simulink model "SimulinkBallbotModel"  (R2017a)
settings: Solver=FixedStepDiscrete  StartTime=0.0  StopTime=10  RelTol=1e-3
libraries: simulink x2
settings Model: FPTRunName=Active  ExtModeTrigDuration=2  Creator=Christopher  LastModifiedBy=Christopher
settings DataIOCC: LimitDataPoints=on  SaveFormat=Array  DSMLogging=off
settings OptimizationCC: DefaultParameterBehavior=Inlined  UseDivisionForNetSlopeComputation=on  UseFloatMulNetSlope=on  InlineInvariantSignals=on  PassReuseOutputArgsAs=Individual arguments  ExpressionDepthLimit=2147483647  ZeroExternalMemoryAtStartup=off  ZeroInternalMemoryAtStartup=off  NoFixptDivByZeroProtection=on  EfficientFloat2IntCast=on  LifeSpan=1  MaxStackSize=64  OptimizeBlockOrder=speed
settings DebuggingCC: UnderspecifiedInitializationDetection=Classic  MergeDetectMultiDrivingBlocksExec=none  ParameterOverflowMsg=warning  ParameterPrecisionLossMsg=none  ParameterTunabilityLossMsg=error  FcnCallInpInsideContextMsg=warning  AllowSymbolicDim=off  StateNameClashWarn=warning  SFUnexpectedBacktrackingDiag=warning  SFNoUnconditionalDefaultTransitionDiag=warning  SFExecutionAtInitializationDiag=none
settings HardwareCC: ProdBitPerInt=16  ProdBitPerPointer=16  ProdBitPerSizeT=16  ProdBitPerPtrDiffT=16  ProdLargestAtomicFloat=None  ProdWordSize=8  ProdHWDeviceType=Atmel->AVR
settings ModelReferenceCC: PropagateSignalLabelsOutOfModel=off
settings SFSimCC: MATLABDynamicMemAlloc=off
settings RTWCC: SystemTargetFile=ert.tlc  HardwareBoard=Arduino Mega 2560  TLCOptions=-aInlineSetEventsForThisBaseRateFcn=TLC_FALSE -aSuppressMultiTaskScheduler=TLC_FALSE -aRateBasedStepFcn=1  GenCodeOnly=on  TemplateMakefile=ert_default_tmf  Description=Embedded Coder  GenerateReport=on  RTWVerbose=off  Toolchain=Arduino AVR  BuildConfiguration=Faster Runs  IncludeHyperlinkInReport=on  LaunchReport=on  GenerateTraceInfo=on  GenerateTraceReport=on  GenerateTraceReportSl=on  GenerateTraceReportSf=on  GenerateTraceReportEml=on  GenerateCodeMetricsReport=on
settings CodeAppCC: ForceParamTrailComments=on  IgnoreCustomStorageClasses=off  OperatorAnnotations=on  SimulinkDataObjDesc=on  SFDataObjDesc=on  MATLABFcnDesc=on  CustomSymbolStrGlobalVar=rt$N$M  CustomSymbolStrType=$N$M  CustomSymbolStrFcn=$N$M$F  CustomSymbolStrMacro=$N$M  InsertBlockDesc=on  MATLABSourceComments=on
settings ERTTargetCC: TargetLangStandard=C99 (ISO)  IncludeMdlTerminateFcn=off  CombineSignalStateStructs=on  SuppressErrorStatus=on  SupportAbsoluteTime=off  SupportNonFinite=off  SupportComplex=off  InlinedParameterPlacement=NonHierarchical  ERTFilePackagingFormat=CompactWithDataFile
settings ConfigComp: CovMetricSettings=dw  CovHtmlReporting=on  CovSaveCumulativeToWorkspaceVar=on  CovSaveSingleToWorkspaceVar=on  CovExternalEMLEnable=off  CovSFcnEnable=off

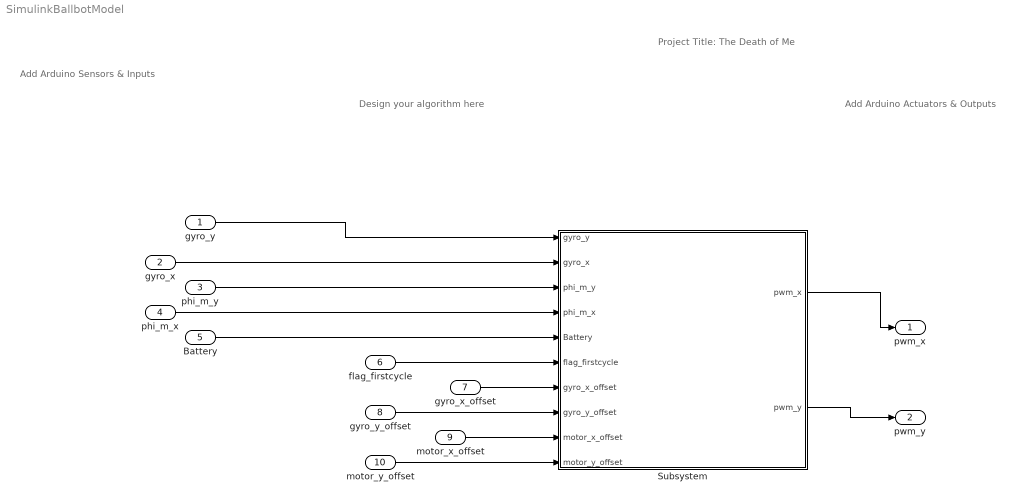
== system SimulinkBallbotModel ==
  note: Project Title: The Death of Me
  note: Add Arduino Sensors & Inputs
  note: Design your algorithm here
  note: Add Arduino Actuators & Outputs
  gyro_y : Inport  OutDataTypeStr=uint16
  gyro_x : Inport  Port=2  OutDataTypeStr=uint16
  phi_m_y : Inport  Port=3  OutDataTypeStr=int32
  phi_m_x : Inport  Port=4  OutDataTypeStr=int32
  Battery : Inport  Port=5  OutDataTypeStr=single
  flag_firstcycle : Inport  Port=6  OutDataTypeStr=boolean
  gyro_x_offset : Inport  Port=7  OutDataTypeStr=single
  gyro_y_offset : Inport  Port=8  OutDataTypeStr=single
  motor_x_offset : Inport  Port=9  OutDataTypeStr=single
  motor_y_offset : Inport  Port=10  OutDataTypeStr=single
  Subsystem : Subsystem
  pwm_x : Outport  OutDataTypeStr=int8
  pwm_y : Outport  Port=2  OutDataTypeStr=int8
  wires:
  phi_m_x/1 -> Subsystem/4(phi_m_x)
  Battery/1 -> Subsystem/5(Battery)
  Subsystem/1(pwm_x) -> pwm_x/1
  Subsystem/2(pwm_y) -> pwm_y/1
  phi_m_y/1 -> Subsystem/3(phi_m_y)
  gyro_x/1 -> Subsystem/2(gyro_x)
  gyro_y/1 -> Subsystem/1(gyro_y)
  flag_firstcycle/1 -> Subsystem/6(flag_firstcycle)
  gyro_x_offset/1 -> Subsystem/7(gyro_x_offset)
  gyro_y_offset/1 -> Subsystem/8(gyro_y_offset)
  motor_x_offset/1 -> Subsystem/9(motor_x_offset)
  motor_y_offset/1 -> Subsystem/10(motor_y_offset)

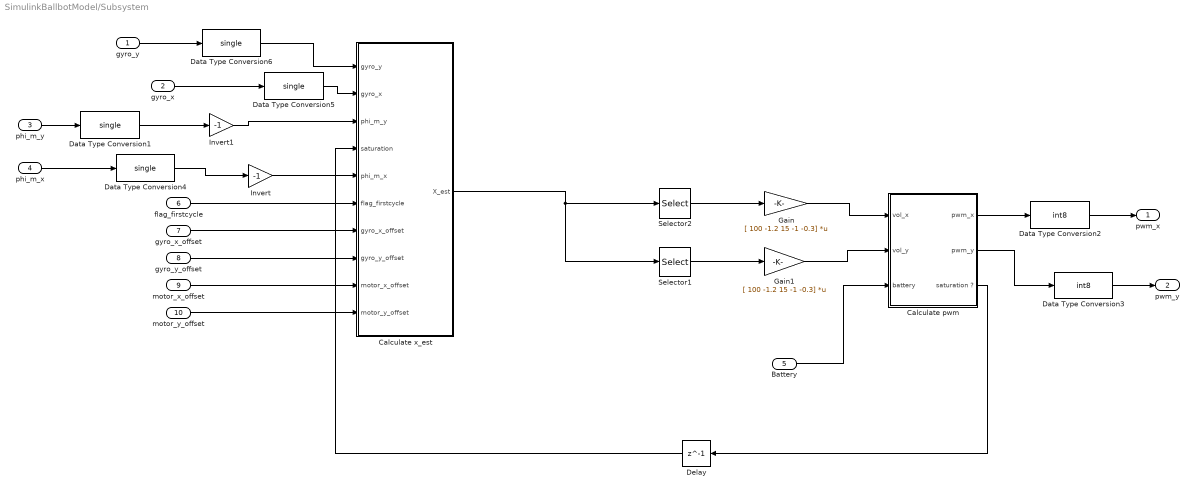
== system SimulinkBallbotModel/Subsystem ==
  gyro_y : Inport
  gyro_x : Inport  Port=2
  phi_m_y : Inport  Port=3  OutDataTypeStr=int32
  phi_m_x : Inport  Port=4  OutDataTypeStr=int32
  Battery : Inport  Port=5  OutDataTypeStr=single
  flag_firstcycle : Inport  Port=6
  gyro_x_offset : Inport  Port=7
  gyro_y_offset : Inport  Port=8
  motor_x_offset : Inport  Port=9
  motor_y_offset : Inport  Port=10
  Calculate pwm : Subsystem
  Calculate x_est : Subsystem
  Data Type Conversion{1,4..6} (4 alike) : DataTypeConversion  OutDataTypeStr=single  RndMeth=Simplest
  Data Type Conversion2 : DataTypeConversion  OutDataTypeStr=int8  RndMeth=Simplest
  Data Type Conversion3 : DataTypeConversion  OutDataTypeStr=int8  RndMeth=Simplest
  Delay : Delay  DelayLength=1  InitialCondition=0
  Gain : Gain  Gain=[ 100 -1.2 15 -1 -0.3]  Multiplication=Matrix(K*u) (u vector)  OutDataTypeStr=single
  Gain1 : Gain  Gain=[ 100 -1.2 15 -1 -0.3]  Multiplication=Matrix(K*u) (u vector)  OutDataTypeStr=single
  Invert : Gain  Gain=-1  OutDataTypeStr=single
  Invert1 : Gain  Gain=-1  OutDataTypeStr=single
  Selector1 : Selector  IndexMode=Zero-based  InputPortWidth=10  IndexOptions=Starting index (dialog)  Indices=5  OutputSizes=5
  Selector2 : Selector  IndexMode=Zero-based  InputPortWidth=10  IndexOptions=Starting index (dialog)  Indices=0  OutputSizes=5
  pwm_x : Outport  OutDataTypeStr=int8
  pwm_y : Outport  Port=2  OutDataTypeStr=int8
  wires:
  Gain1/1 -> Calculate pwm/2(vol_y)
  Calculate x_est/1(X_est) -> Selector1/1, Selector2/1
  Gain/1 -> Calculate pwm/1(vol_x)
  gyro_x/1 -> Data Type Conversion5/1
  Calculate pwm/1(pwm_x) -> Data Type Conversion2/1
  phi_m_x/1 -> Data Type Conversion4/1
  Delay/1 -> Calculate x_est/4(saturation)
  Calculate pwm/2(pwm_y) -> Data Type Conversion3/1
  phi_m_y/1 -> Data Type Conversion1/1
  Battery/1 -> Calculate pwm/3(battery)
  Selector2/1 -> Gain/1
  Calculate pwm/3(saturation ?) -> Delay/1
  Selector1/1 -> Gain1/1
  gyro_y/1 -> Data Type Conversion6/1
  flag_firstcycle/1 -> Calculate x_est/6(flag_firstcycle)
  gyro_x_offset/1 -> Calculate x_est/7(gyro_x_offset)
  gyro_y_offset/1 -> Calculate x_est/8(gyro_y_offset)
  motor_x_offset/1 -> Calculate x_est/9(motor_x_offset)
  motor_y_offset/1 -> Calculate x_est/10(motor_y_offset)
  Data Type Conversion2/1 -> pwm_x/1
  Data Type Conversion3/1 -> pwm_y/1
  Data Type Conversion6/1 -> Calculate x_est/1(gyro_y)
  Data Type Conversion5/1 -> Calculate x_est/2(gyro_x)
  Data Type Conversion1/1 -> Invert1/1
  Data Type Conversion4/1 -> Invert/1
  Invert/1 -> Calculate x_est/5(phi_m_x)
  Invert1/1 -> Calculate x_est/3(phi_m_y)

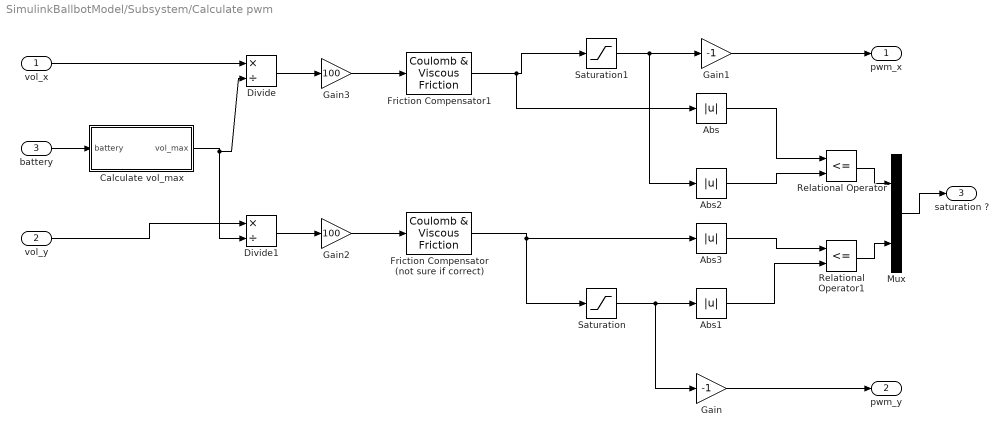
== system SimulinkBallbotModel/Subsystem/Calculate pwm ==
  vol_x : Inport  OutDataTypeStr=single
  vol_y : Inport  Port=2  OutDataTypeStr=single
  battery : Inport  Port=3  OutDataTypeStr=single
  Abs{,1..3} (4 alike) : Abs
  Calculate vol_max : Subsystem
  Divide : Product  Inputs=*/  OutDataTypeStr=single
  Divide1 : Product  Inputs=*/  OutDataTypeStr=single
  Friction Compensator (not sure if correct) : simulink/Discontinuities/Coulomb & Viscous Friction  offset=0  gain=1
      settings: SourceProductName=Simulink
  Friction Compensator1 : simulink/Discontinuities/Coulomb & Viscous Friction  offset=0  gain=1
      settings: SourceProductName=Simulink
  Gain : Gain  Gain=-1  OutDataTypeStr=single  RndMeth=Simplest
  Gain1 : Gain  Gain=-1  OutDataTypeStr=single  RndMeth=Simplest
  Gain2 : Gain  Gain=100  OutDataTypeStr=single
  Gain3 : Gain  Gain=100  OutDataTypeStr=single
  Mux : Mux  Inputs=2
  Relational Operator : RelationalOperator  Operator=<=  OutDataTypeStr=boolean  RndMeth=Simplest
  Relational Operator1 : RelationalOperator  Operator=<=  OutDataTypeStr=boolean  RndMeth=Simplest
  Saturation : Saturate  UpperLimit=100  LowerLimit=-100  OutDataTypeStr=single
  Saturation1 : Saturate  UpperLimit=100  LowerLimit=-100  OutDataTypeStr=single
  pwm_x : Outport  OutDataTypeStr=single
  pwm_y : Outport  Port=2  OutDataTypeStr=single
  saturation ? : Outport  Port=3  OutDataTypeStr=boolean
  wires:
  battery/1 -> Calculate vol_max/1(battery)
  Gain/1 -> pwm_y/1
  Gain1/1 -> pwm_x/1
  Mux/1 -> saturation ?/1
  Relational Operator/1 -> Mux/1
  Relational Operator1/1 -> Mux/2
  Abs3/1 -> Relational Operator1/1
  Abs1/1 -> Relational Operator1/2
  Abs2/1 -> Relational Operator/2
  Abs/1 -> Relational Operator/1
  Saturation/1 -> Gain/1, Abs1/1
  Saturation1/1 -> Abs2/1, Gain1/1
  vol_x/1 -> Divide/1
  vol_y/1 -> Divide1/1
  Calculate vol_max/1(vol_max) -> Divide/2, Divide1/2
  Divide/1 -> Gain3/1
  Divide1/1 -> Gain2/1
  Gain2/1 -> Friction Compensator (not sure if correct)/1
  Gain3/1 -> Friction Compensator1/1
  Friction Compensator1/1 -> Abs/1, Saturation1/1
  Friction Compensator (not sure if correct)/1 -> Abs3/1, Saturation/1

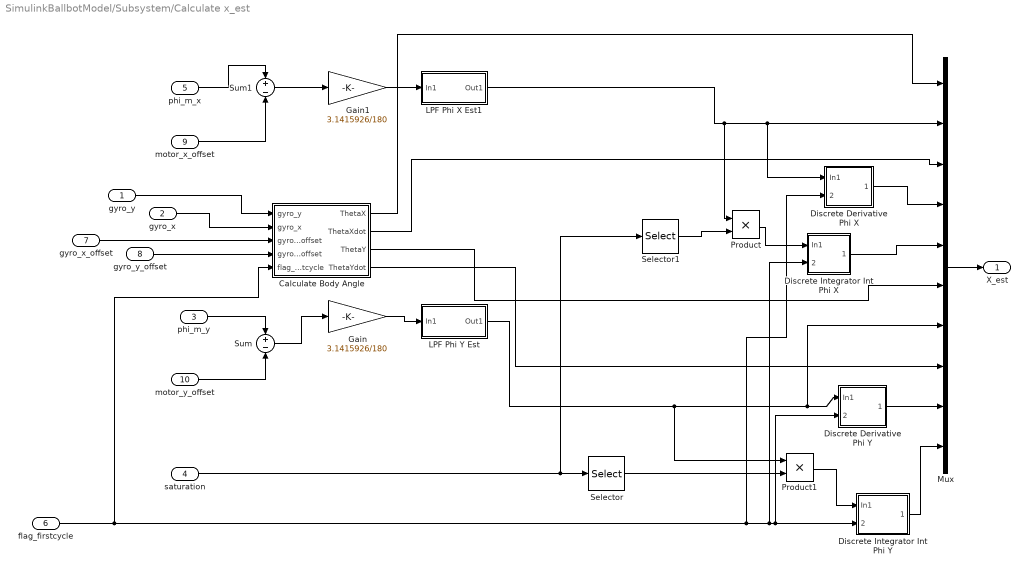
== system SimulinkBallbotModel/Subsystem/Calculate x_est ==
  gyro_y : Inport  OutDataTypeStr=single
  gyro_x : Inport  Port=2  OutDataTypeStr=single
  phi_m_y : Inport  Port=3
  saturation : Inport  Port=4  OutDataTypeStr=boolean
  phi_m_x : Inport  Port=5
  flag_firstcycle : Inport  Port=6
  gyro_x_offset : Inport  Port=7
  gyro_y_offset : Inport  Port=8
  motor_x_offset : Inport  Port=9
  motor_y_offset : Inport  Port=10
  Calculate Body Angle : Subsystem
  Discrete Derivative Phi X : Subsystem  TreatAsAtomicUnit=on
  Discrete Derivative Phi Y : Subsystem  TreatAsAtomicUnit=on
  Discrete Integrator Int Phi X : Subsystem  TreatAsAtomicUnit=on
  Discrete Integrator Int Phi Y : Subsystem  TreatAsAtomicUnit=on
  Gain : Gain  Gain=3.1415926/180  OutDataTypeStr=single
  Gain1 : Gain  Gain=3.1415926/180  OutDataTypeStr=single
  LPF Phi X Est1 : Subsystem
  LPF Phi Y Est : Subsystem
  Mux : Mux  Inputs=10
  Product : Product
  Product1 : Product  OutDataTypeStr=single
  Selector : Selector  IndexMode=Zero-based  InputPortWidth=2  IndexOptions=Starting index (dialog)  Indices=1  OutputSizes=1
  Selector1 : Selector  IndexMode=Zero-based  InputPortWidth=2  IndexOptions=Starting index (dialog)  Indices=0  OutputSizes=1
  Sum : Sum  Inputs=+-
  Sum1 : Sum  Inputs=+-  AccumDataTypeStr=uint8
  X_est : Outport  OutDataTypeStr=single
  wires:
  Mux/1 -> X_est/1
  Product/1 -> Discrete Integrator Int Phi X/1(In1)
  Discrete Integrator Int Phi Y/1(Out1) -> Mux/10
  phi_m_y/1 -> Sum/1
  Discrete Integrator Int Phi X/1(Out1) -> Mux/5
  saturation/1 -> Selector1/1, Selector/1
  Product1/1 -> Discrete Integrator Int Phi Y/1(In1)
  Discrete Derivative Phi Y/1(Out1) -> Mux/9
  Calculate Body Angle/4(ThetaYdot) -> Mux/8
  Sum/1 -> Gain/1
  LPF Phi Y Est/1(Out1) -> Product1/1, Mux/7, Discrete Derivative Phi Y/1(In1)
  Gain1/1 -> LPF Phi X Est1/1(In1)
  Sum1/1 -> Gain1/1
  Discrete Derivative Phi X/1(Out1) -> Mux/4
  Selector1/1 -> Product/2
  Selector/1 -> Product1/2
  Gain/1 -> LPF Phi Y Est/1(In1)
  gyro_x/1 -> Calculate Body Angle/2(gyro_x)
  phi_m_x/1 -> Sum1/1
  Calculate Body Angle/2(ThetaXdot) -> Mux/3
  Calculate Body Angle/3(ThetaY) -> Mux/6
  gyro_y/1 -> Calculate Body Angle/1(gyro_y)
  LPF Phi X Est1/1(Out1) -> Product/1, Discrete Derivative Phi X/1(In1), Mux/2
  Calculate Body Angle/1(ThetaX) -> Mux/1
  motor_x_offset/1 -> Sum1/2
  motor_y_offset/1 -> Sum/2
  flag_firstcycle/1 -> Calculate Body Angle/5(flag_firstcycle), Discrete Integrator Int Phi X/2(flag_firstcycle), Discrete Derivative Phi Y/2(flag_firstcycle), Discrete Integrator Int Phi Y/2(flag_firstcycle), Discrete Derivative Phi X/2(flag_firstcycle)
  gyro_x_offset/1 -> Calculate Body Angle/3(gyro_x_offset)
  gyro_y_offset/1 -> Calculate Body Angle/4(gyro_y_offset)

== system SimulinkBallbotModel/Subsystem/Calculate pwm/Calculate vol_max ==
  battery : Inport
  Constant : Constant  Value=0.625  OutDataTypeStr=single
  Gain : Gain  Gain=.001089  OutDataTypeStr=single  RndMeth=Simplest
  Sum : Sum  Inputs=+-
  vol_max : Outport
  wires:
  battery/1 -> Gain/1
  Gain/1 -> Sum/1
  Constant/1 -> Sum/2
  Sum/1 -> vol_max/1

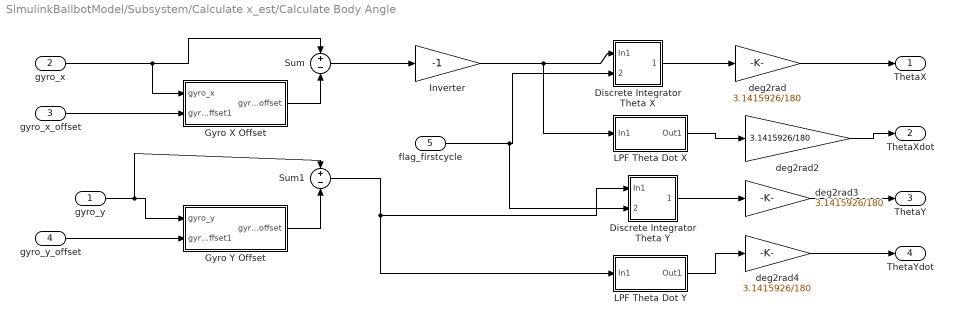
== system SimulinkBallbotModel/Subsystem/Calculate x_est/Calculate Body Angle ==
  gyro_y : Inport  OutDataTypeStr=single
  gyro_x : Inport  Port=2  OutDataTypeStr=single
  gyro_x_offset : Inport  Port=3  OutDataTypeStr=single
  gyro_y_offset : Inport  Port=4  OutDataTypeStr=single
  flag_firstcycle : Inport  Port=5  OutDataTypeStr=boolean
  Discrete Integrator Theta Y : Subsystem  TreatAsAtomicUnit=on
  Discrete Integrator Theta X : Subsystem  TreatAsAtomicUnit=on
  Gyro X Offset : Subsystem
  Gyro Y Offset : Subsystem
  Inverter : Gain  Gain=-1  OutDataTypeStr=single
  LPF Theta Dot X : Subsystem
  LPF Theta Dot Y : Subsystem
  Sum : Sum  Inputs=+-
  Sum1 : Sum  Inputs=+-
  deg2rad{,2..4} (4 alike) : Gain  Gain=3.1415926/180  OutDataTypeStr=single
  ThetaX : Outport  OutDataTypeStr=single
  ThetaXdot : Outport  Port=2  OutDataTypeStr=single
  ThetaY : Outport  Port=3  OutDataTypeStr=single
  ThetaYdot : Outport  Port=4  OutDataTypeStr=single
  wires:
  deg2rad/1 -> ThetaX/1
  deg2rad4/1 -> ThetaYdot/1
  deg2rad3/1 -> ThetaY/1
  deg2rad2/1 -> ThetaXdot/1
  Gyro Y Offset/1(gyro_y_offset) -> Sum1/2
  Sum/1 -> Inverter/1
  Gyro X Offset/1(gyro_x_offset) -> Sum/2
  Discrete Integrator Theta X/1(Out1) -> deg2rad/1
  Discrete Integrator Theta Y/1(Out1) -> deg2rad3/1
  LPF Theta Dot X/1(Out1) -> deg2rad2/1
  LPF Theta Dot Y/1(Out1) -> deg2rad4/1
  Sum1/1 -> Discrete Integrator Theta Y/1(In1), LPF Theta Dot Y/1(In1)
  Inverter/1 -> LPF Theta Dot X/1(In1), Discrete Integrator Theta X/1(In1)
  gyro_x_offset/1 -> Gyro X Offset/2(gyro_x_offset1)
  gyro_y_offset/1 -> Gyro Y Offset/2(gyro_y_offset1)
  flag_firstcycle/1 -> Discrete Integrator Theta Y/2(flag_firstcycle), Discrete Integrator Theta X/2(flag_firstcycle)
  gyro_x/1 -> Gyro X Offset/1(gyro_x), Sum/1
  gyro_y/1 -> Sum1/1, Gyro Y Offset/1(gyro_y)

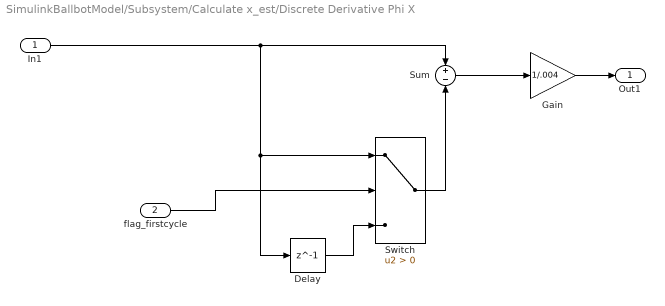
== system SimulinkBallbotModel/Subsystem/Calculate x_est/Discrete Derivative Phi X ==
  In1 : Inport
  flag_firstcycle : Inport  Port=2  OutDataTypeStr=boolean
  Delay : Delay  DelayLength=1  InitialCondition=0
  Gain : Gain  Gain=1/.004  OutDataTypeStr=single
  Sum : Sum  Inputs=+-
  Switch : Switch  Criteria=u2 > Threshold  OutDataTypeStr=single
  Out1 : Outport  OutDataTypeStr=single
  wires:
  Gain/1 -> Out1/1
  Switch/1 -> Sum/2
  In1/1 -> Delay/1, Switch/1, Sum/1
  Sum/1 -> Gain/1
  Delay/1 -> Switch/3
  flag_firstcycle/1 -> Switch/2

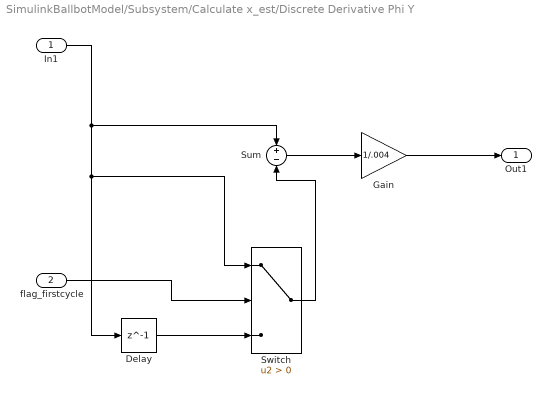
== system SimulinkBallbotModel/Subsystem/Calculate x_est/Discrete Derivative Phi Y ==
  In1 : Inport  OutDataTypeStr=single
  flag_firstcycle : Inport  Port=2
  Delay : Delay  DelayLength=1  InitialCondition=0
  Gain : Gain  Gain=1/.004  OutDataTypeStr=single
  Sum : Sum  Inputs=+-
  Switch : Switch  Criteria=u2 > Threshold  OutDataTypeStr=single
  Out1 : Outport  OutDataTypeStr=single
  wires:
  Sum/1 -> Gain/1
  Gain/1 -> Out1/1
  In1/1 -> Delay/1, Switch/1, Sum/1
  Delay/1 -> Switch/3
  Switch/1 -> Sum/2
  flag_firstcycle/1 -> Switch/2

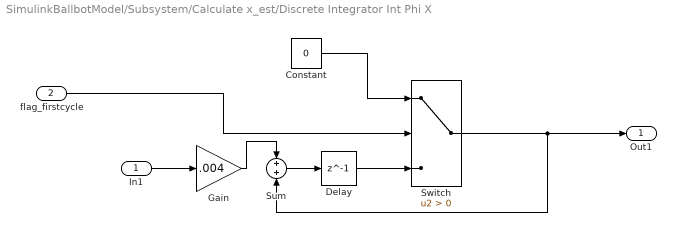
== system SimulinkBallbotModel/Subsystem/Calculate x_est/Discrete Integrator Int Phi X ==
  In1 : Inport  OutDataTypeStr=single
  flag_firstcycle : Inport  Port=2
  Constant : Constant  Value=0  OutDataTypeStr=single
  Delay : Delay  DelayLength=1  InitialCondition=0
  Gain : Gain  Gain=.004  OutDataTypeStr=single  RndMeth=Simplest
  Sum : Sum
  Switch : Switch  Criteria=u2 > Threshold  OutDataTypeStr=single
  Out1 : Outport  OutDataTypeStr=single
  wires:
  flag_firstcycle/1 -> Switch/2
  Delay/1 -> Switch/3
  In1/1 -> Gain/1
  Gain/1 -> Sum/1
  Sum/1 -> Delay/1
  Switch/1 -> Sum/2, Out1/1
  Constant/1 -> Switch/1

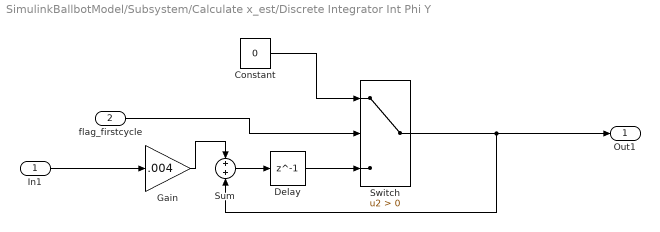
== system SimulinkBallbotModel/Subsystem/Calculate x_est/Discrete Integrator Int Phi Y ==
  In1 : Inport  OutDataTypeStr=single
  flag_firstcycle : Inport  Port=2  OutDataTypeStr=boolean
  Constant : Constant  Value=0  OutDataTypeStr=single
  Delay : Delay  DelayLength=1  InitialCondition=0
  Gain : Gain  Gain=.004  OutDataTypeStr=single  RndMeth=Simplest
  Sum : Sum
  Switch : Switch  Criteria=u2 > Threshold  OutDataTypeStr=single
  Out1 : Outport  OutDataTypeStr=single
  wires:
  Switch/1 -> Sum/2, Out1/1
  Delay/1 -> Switch/3
  flag_firstcycle/1 -> Switch/2
  Sum/1 -> Delay/1
  Constant/1 -> Switch/1
  Gain/1 -> Sum/1
  In1/1 -> Gain/1

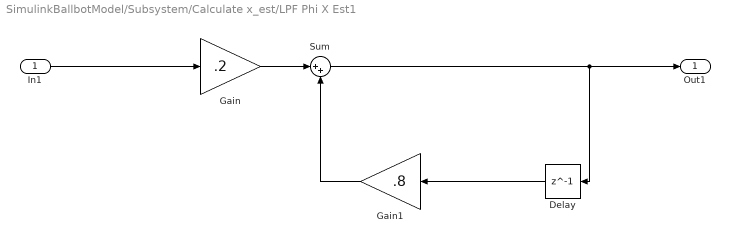
== system SimulinkBallbotModel/Subsystem/Calculate x_est/LPF Phi X Est1 ==
  In1 : Inport  OutDataTypeStr=single
  Delay : Delay  DelayLength=1  InitialCondition=0
  Gain : Gain  Gain=.2  OutDataTypeStr=single
  Gain1 : Gain  Gain=.8  OutDataTypeStr=single
  Sum : Sum  Inputs=|++
  Out1 : Outport  OutDataTypeStr=single
  wires:
  In1/1 -> Gain/1
  Gain1/1 -> Sum/2
  Gain/1 -> Sum/1
  Sum/1 -> Delay/1, Out1/1
  Delay/1 -> Gain1/1

== system SimulinkBallbotModel/Subsystem/Calculate x_est/LPF Phi Y Est ==
  In1 : Inport
  Delay : Delay  DelayLength=1  InitialCondition=0
  Gain : Gain  Gain=.2  OutDataTypeStr=single
  Gain1 : Gain  Gain=.8  OutDataTypeStr=single
  Sum : Sum  Inputs=|++
  Out1 : Outport  OutDataTypeStr=single
  wires:
  Sum/1 -> Out1/1, Delay/1
  Gain1/1 -> Sum/2
  Delay/1 -> Gain1/1
  Gain/1 -> Sum/1
  In1/1 -> Gain/1

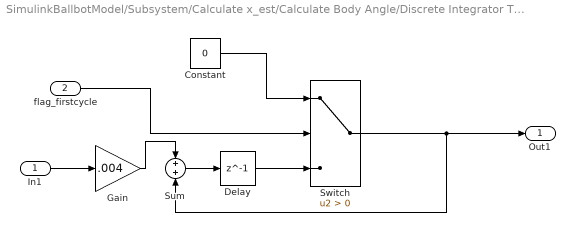
== system SimulinkBallbotModel/Subsystem/Calculate x_est/Calculate Body Angle/Discrete Integrator Theta Y ==
  In1 : Inport  OutDataTypeStr=single
  flag_firstcycle : Inport  Port=2  OutDataTypeStr=boolean
  Constant : Constant  Value=0  OutDataTypeStr=single
  Delay : Delay  DelayLength=1  InitialCondition=0
  Gain : Gain  Gain=.004  OutDataTypeStr=single
  Sum : Sum
  Switch : Switch  Criteria=u2 > Threshold  OutDataTypeStr=single
  Out1 : Outport  OutDataTypeStr=single
  wires:
  flag_firstcycle/1 -> Switch/2
  Delay/1 -> Switch/3
  In1/1 -> Gain/1
  Gain/1 -> Sum/1
  Sum/1 -> Delay/1
  Switch/1 -> Sum/2, Out1/1
  Constant/1 -> Switch/1

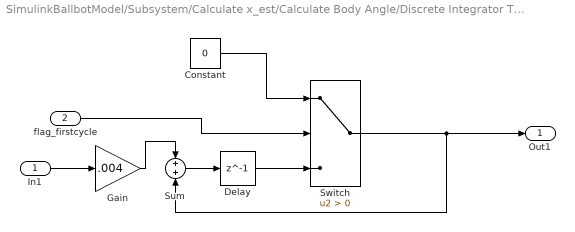
== system SimulinkBallbotModel/Subsystem/Calculate x_est/Calculate Body Angle/Discrete Integrator Theta X ==
  In1 : Inport
  flag_firstcycle : Inport  Port=2  OutDataTypeStr=boolean
  Constant : Constant  Value=0  OutDataTypeStr=single
  Delay : Delay  DelayLength=1  InitialCondition=0
  Gain : Gain  Gain=.004  OutDataTypeStr=single
  Sum : Sum
  Switch : Switch  Criteria=u2 > Threshold  OutDataTypeStr=single
  Out1 : Outport  OutDataTypeStr=single
  wires:
  flag_firstcycle/1 -> Switch/2
  Delay/1 -> Switch/3
  In1/1 -> Gain/1
  Gain/1 -> Sum/1
  Sum/1 -> Delay/1
  Switch/1 -> Sum/2, Out1/1
  Constant/1 -> Switch/1

== system SimulinkBallbotModel/Subsystem/Calculate x_est/Calculate Body Angle/Gyro X Offset ==
  gyro_x : Inport  OutDataTypeStr=single
  gyro_x_offset1 : Inport  Port=2  OutDataTypeStr=single
  1-a_gd : Gain  Gain=.001  OutDataTypeStr=single
  Sum : Sum  Inputs=|++
  a_gd : Gain  Gain=.999  OutDataTypeStr=single
  gyro_x_offset : Outport  OutDataTypeStr=single
  wires:
  gyro_x/1 -> 1-a_gd/1
  1-a_gd/1 -> Sum/2
  Sum/1 -> gyro_x_offset/1
  a_gd/1 -> Sum/1
  gyro_x_offset1/1 -> a_gd/1

== system SimulinkBallbotModel/Subsystem/Calculate x_est/Calculate Body Angle/Gyro Y Offset ==
  gyro_y : Inport  OutDataTypeStr=single
  gyro_y_offset1 : Inport  Port=2  OutDataTypeStr=single
  1-a_gd : Gain  Gain=.001  OutDataTypeStr=single
  Sum : Sum  Inputs=|++
  a_gd : Gain  Gain=.999  OutDataTypeStr=uint8
  gyro_y_offset : Outport  OutDataTypeStr=single
  wires:
  a_gd/1 -> Sum/1
  1-a_gd/1 -> Sum/2
  gyro_y_offset1/1 -> a_gd/1
  gyro_y/1 -> 1-a_gd/1
  Sum/1 -> gyro_y_offset/1

== system SimulinkBallbotModel/Subsystem/Calculate x_est/Calculate Body Angle/LPF Theta Dot X ==
  In1 : Inport  OutDataTypeStr=single
  1-a_gyro : Gain  Gain=.75  OutDataTypeStr=single
  Delay : Delay  DelayLength=1  InitialCondition=0
  Sum : Sum  Inputs=|++
  a_gyro : Gain  Gain=.25  OutDataTypeStr=single
  Out1 : Outport  OutDataTypeStr=single
  wires:
  In1/1 -> 1-a_gyro/1
  a_gyro/1 -> Sum/2
  1-a_gyro/1 -> Sum/1
  Sum/1 -> Delay/1, Out1/1
  Delay/1 -> a_gyro/1

== system SimulinkBallbotModel/Subsystem/Calculate x_est/Calculate Body Angle/LPF Theta Dot Y ==
  In1 : Inport  OutDataTypeStr=single
  1-a_gyro : Gain  Gain=.75  OutDataTypeStr=single
  Delay : Delay  DelayLength=1  InitialCondition=0
  Sum : Sum  Inputs=|++
  a_gyro : Gain  Gain=.25  OutDataTypeStr=single
  Out1 : Outport  OutDataTypeStr=single
  wires:
  In1/1 -> 1-a_gyro/1
  a_gyro/1 -> Sum/2
  1-a_gyro/1 -> Sum/1
  Sum/1 -> Delay/1, Out1/1
  Delay/1 -> a_gyro/1
